simulink model "b_r309c_med"  (Simulink 6.2)
settings: Solver=ode45  StartTime=0.0  StopTime=1030.0  RelTol=1e-3
undefined symbols (not defined in the file): ant_bits, BEE2_usr, blockCountBits, blockRowBits, cmult_4bit_em
libraries: xbsIndex_r3 x2808, xps_library x97, casper_library x84
(part 3 of 20)

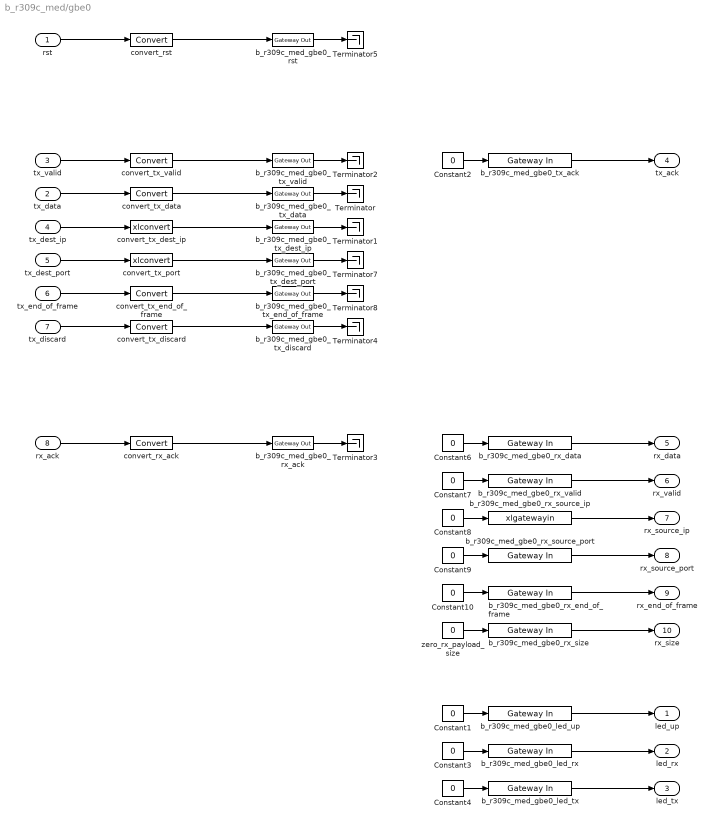
== system b_r309c_med/gbe0 ==
  rst : Inport  Port=1  LatchInput=off
  tx_data : Inport  Port=2  LatchInput=off
  tx_valid : Inport  Port=3  LatchInput=off
  tx_dest_ip : Inport  Port=4  LatchInput=off
  tx_dest_port : Inport  Port=5  LatchInput=off
  tx_end_of_frame : Inport  Port=6  LatchInput=off
  tx_discard : Inport  Port=7  LatchInput=off
  rx_ack : Inport  Port=8  LatchInput=off
  Constant{1..4,6..10} (9 alike) : Constant  Value=0
  Terminator{,1..5,7..8} (8 alike) : Terminator
  b_r309c_med_gbe0_led_rx : xbsIndex_r3/Gateway In  arith_type=Boolean  n_bits=1  bin_pt=0  quantization=Truncate  overflow=Wrap  period=1  timing_constraint=None  locs_specified=off  LOCs={}  needs_fixed_name=off  dbl_ovrd=off  show_param=off
      settings: xl_area=[0, 0, 0, 0, 0, 0, 0]
  b_r309c_med_gbe0_led_tx : xbsIndex_r3/Gateway In  arith_type=Boolean  n_bits=1  bin_pt=0  quantization=Truncate  overflow=Wrap  period=1  timing_constraint=None  locs_specified=off  LOCs={}  needs_fixed_name=off  dbl_ovrd=off  show_param=off
      settings: xl_area=[0, 0, 0, 0, 0, 0, 0]
  b_r309c_med_gbe0_led_up : xbsIndex_r3/Gateway In  arith_type=Boolean  n_bits=1  bin_pt=0  quantization=Truncate  overflow=Wrap  period=1  timing_constraint=None  locs_specified=off  LOCs={}  needs_fixed_name=off  dbl_ovrd=off  show_param=off
      settings: xl_area=[0, 0, 0, 0, 0, 0, 0]
  b_r309c_med_gbe0_rst : xbsIndex_r3/Gateway Out  output_type=Double  nbits=8  bin_pt=6  arith_type=Boolean  quantization=Truncate  overflow=Wrap  hdl_port=on  timing_constraint=None  locs_specified=off  LOCs={}  needs_fixed_name=off  show_param=off
      settings: xl_area=[0, 0, 0, 0, 0, 0, 0]
  b_r309c_med_gbe0_rx_ack : xbsIndex_r3/Gateway Out  output_type=Double  nbits=8  bin_pt=6  arith_type=Boolean  quantization=Truncate  overflow=Wrap  hdl_port=on  timing_constraint=None  locs_specified=off  LOCs={}  needs_fixed_name=off  show_param=off
      settings: xl_area=[0, 0, 0, 0, 0, 0, 0]
  b_r309c_med_gbe0_rx_data : xbsIndex_r3/Gateway In  arith_type=Unsigned  n_bits=64  bin_pt=0  quantization=Truncate  overflow=Wrap  period=1  timing_constraint=None  locs_specified=off  LOCs={}  needs_fixed_name=off  dbl_ovrd=off  show_param=off
      settings: xl_area=[0, 0, 0, 0, 0, 0, 0]
  b_r309c_med_gbe0_rx_end_of_frame : xbsIndex_r3/Gateway In  arith_type=Boolean  n_bits=1  bin_pt=0  quantization=Truncate  overflow=Wrap  period=1  timing_constraint=None  locs_specified=off  LOCs={}  needs_fixed_name=off  dbl_ovrd=off  show_param=off
      settings: xl_area=[0, 0, 0, 0, 0, 0, 0]
  b_r309c_med_gbe0_rx_size : xbsIndex_r3/Gateway In  arith_type=Unsigned  n_bits=16  bin_pt=0  quantization=Truncate  overflow=Wrap  period=1  timing_constraint=None  locs_specified=off  LOCs={}  needs_fixed_name=off  dbl_ovrd=off  show_param=off
      settings: xl_area=[0, 0, 0, 0, 0, 0, 0]
  b_r309c_med_gbe0_rx_source_ip : S-Function  AncestorBlock=xbsIndex_r3/Gateway In  FunctionName=xlgatewayin  Parameters="arith_type, n_bits, bin_pt, quantization, overflow,  gcb, period, dbl_ovrd, locs_specified, LOCs, timing_constraint, simulinkPeriod, designRoot, 0"  mask(Xilinx Gateway In){arith_type=Unsigned, n_bits=32, bin_pt=0, quantization=Truncate, overflow=Wrap, period=1, timing_constraint=None, locs_specified=off, LOCs={}, needs_fixed_name=off, dbl_ovrd=off, show_param=off, xl_area=[0, 0, 0, 0, 0, 0, 0], xl_use_area=off}
      mask prompts: arith_type "Output Data Type"; n_bits "Number of Bits"; bin_pt "Binary Point"; period "Sample Period"; timing_constraint "IOB Timing Constraint"; locs_specified "Specify IOB Location Constraints"; LOCs "IOB Pad Locations (specify as cell array {'MSB', ..., 'LSB'})"; needs_fixed_name "Do Not Prepend Hierarchy to Port Name"; dbl_ovrd "Override with Double"; show_param "---------------------- Show Implementation Parameters -----------------------------------------------------------------------------------"; xl_area "FPGA Area [Slices, FFs, BRAMs, LUTs, IOBs, Emb. Mults, TBUFs]"; xl_use_area "Use Area Above For Estimation"
      mask help:
      | Gateway in block.  Converts inputs of type Simulink integer, double and fixed point to  Xilinx fixed point type.
      |
      | Hardware notes:  In hardware these blocks become top level input ports.
      mask init:
      | [designRoot, family, part, speed, package, simulinkPeriod, sysclkPeriod, dbl_ovrd, trimVbit] = xlSysgenSettings(gcb,1,0);
      | trimVbit = 1;
      | [bg,fg] = xlcmap('IO',dbl_ovrd);
      | iPos = get_param(gcb,'Position');
      | iWidth=iPos(3)-iPos(1); iHeight=iPos(4)-iPos(2);
      | iCx=iWidth/2;
      | iCy=iHeight/2;
      | [logoX, logoY] = xlogo(iPos);
      mask Help: eval('xlWeb(xlhtmldoclink(''Gateway In''))');
      mask StyleString: popup(Boolean|Unsigned|Signed  (2's comp)),edit,edit,popup(Truncate|Round  (unbiased: +/- Inf)),popup(Wrap|Saturate|Flag as Error),edit,popup(None|Data Rate|Data Rate;  Set 'FAST' Attribute),checkbox,edit,checkbox,checkbox,checkbox,edit,checkbox
      mask CallbackString: xlgatewayinCallback|||||||xlgatewayinCallback||||xlShowIPCallback||
      mask Display:
      | patch([0 iWidth iWidth 0],[0 0 iHeight iHeight] , bg);
      | patch(logoX,logoY , fg);
      | port_label('input',1,'dbl');
      | port_label('output',1,'fpt');
      | 
      | ;plot([0 0 iWidth iWidth 0], [0 iHeight iHeight 0 0]);
  b_r309c_med_gbe0_rx_source_port : xbsIndex_r3/Gateway In  arith_type=Unsigned  n_bits=16  bin_pt=0  quantization=Truncate  overflow=Wrap  period=1  timing_constraint=None  locs_specified=off  LOCs={}  needs_fixed_name=off  dbl_ovrd=off  show_param=off
      settings: xl_area=[0, 0, 0, 0, 0, 0, 0]
  b_r309c_med_gbe0_rx_valid : xbsIndex_r3/Gateway In  arith_type=Boolean  n_bits=1  bin_pt=0  quantization=Truncate  overflow=Wrap  period=1  timing_constraint=None  locs_specified=off  LOCs={}  needs_fixed_name=off  dbl_ovrd=off  show_param=off
      settings: xl_area=[0, 0, 0, 0, 0, 0, 0]
  b_r309c_med_gbe0_tx_ack : xbsIndex_r3/Gateway In  arith_type=Boolean  n_bits=1  bin_pt=0  quantization=Truncate  overflow=Wrap  period=1  timing_constraint=None  locs_specified=off  LOCs={}  needs_fixed_name=off  dbl_ovrd=off  show_param=off
      settings: xl_area=[0, 0, 0, 0, 0, 0, 0]
  b_r309c_med_gbe0_tx_data : xbsIndex_r3/Gateway Out  output_type=Double  nbits=8  bin_pt=6  arith_type=Boolean  quantization=Truncate  overflow=Wrap  hdl_port=on  timing_constraint=None  locs_specified=off  LOCs={}  needs_fixed_name=off  show_param=off
      settings: xl_area=[0, 0, 0, 0, 0, 0, 0]
  b_r309c_med_gbe0_tx_dest_ip : xbsIndex_r3/Gateway Out  output_type=Double  nbits=8  bin_pt=6  arith_type=Boolean  quantization=Truncate  overflow=Wrap  hdl_port=on  timing_constraint=None  locs_specified=off  LOCs={}  needs_fixed_name=off  show_param=off
      settings: xl_area=[0, 0, 0, 0, 0, 0, 0]
  b_r309c_med_gbe0_tx_dest_port : xbsIndex_r3/Gateway Out  output_type=Double  nbits=8  bin_pt=6  arith_type=Boolean  quantization=Truncate  overflow=Wrap  hdl_port=on  timing_constraint=None  locs_specified=off  LOCs={}  needs_fixed_name=off  show_param=off
      settings: xl_area=[0, 0, 0, 0, 0, 0, 0]
  b_r309c_med_gbe0_tx_discard : xbsIndex_r3/Gateway Out  output_type=Double  nbits=8  bin_pt=6  arith_type=Boolean  quantization=Truncate  overflow=Wrap  hdl_port=on  timing_constraint=None  locs_specified=off  LOCs={}  needs_fixed_name=off  show_param=off
      settings: xl_area=[0, 0, 0, 0, 0, 0, 0]
  b_r309c_med_gbe0_tx_end_of_frame : xbsIndex_r3/Gateway Out  output_type=Double  nbits=8  bin_pt=6  arith_type=Boolean  quantization=Truncate  overflow=Wrap  hdl_port=on  timing_constraint=None  locs_specified=off  LOCs={}  needs_fixed_name=off  show_param=off
      settings: xl_area=[0, 0, 0, 0, 0, 0, 0]
  b_r309c_med_gbe0_tx_valid : xbsIndex_r3/Gateway Out  output_type=Double  nbits=8  bin_pt=6  arith_type=Boolean  quantization=Truncate  overflow=Wrap  hdl_port=on  timing_constraint=None  locs_specified=off  LOCs={}  needs_fixed_name=off  show_param=off
      settings: xl_area=[0, 0, 0, 0, 0, 0, 0]
  convert_rst : xbsIndex_r3/Convert  arith_type=Boolean  n_bits=64  bin_pt=0  quantization=Truncate  overflow=Wrap  latency=0  explicit_period=off  period=1  dbl_ovrd=off  show_param=off  inserted_by_tool=off  pipeline=off
      settings: xl_area=[0, 0, 0, 0, 0, 0, 0]
  convert_rx_ack : xbsIndex_r3/Convert  arith_type=Boolean  n_bits=64  bin_pt=0  quantization=Truncate  overflow=Wrap  latency=0  explicit_period=off  period=1  dbl_ovrd=off  show_param=off  inserted_by_tool=off  pipeline=off
      settings: xl_area=[0, 0, 0, 0, 0, 0, 0]
  convert_tx_data : xbsIndex_r3/Convert  arith_type=Unsigned  n_bits=64  bin_pt=0  quantization=Truncate  overflow=Wrap  latency=0  explicit_period=off  period=1  dbl_ovrd=off  show_param=off  inserted_by_tool=off  pipeline=off
      settings: xl_area=[0, 0, 0, 0, 0, 0, 0]
  convert_tx_dest_ip : S-Function  AncestorBlock=xbsIndex_r3/Convert  FunctionName=xlconvert  Parameters=sfcn_mwsv__  mask(Xilinx Converter Block){arith_type=Unsigned, n_bits=32, bin_pt=0, quantization=Truncate, overflow=Wrap, latency=0, explicit_period=off, period=1, dbl_ovrd=off, show_param=off, inserted_by_tool=off, pipeline=off, xl_area=[0, 0, 0, 0, 0, 0, 0], xl_use_area=off}
      mask prompts: arith_type "Output Type"; n_bits "Number of Bits"; bin_pt "Binary Point"; quantization "Quantization Behavior"; overflow "Overflow Behavior"; explicit_period "Use Explicit Sample Period"; period "Sample Period"; dbl_ovrd "Override with Doubles"; show_param "---------------------- Show Implementation Parameters -----------------------------------------------------------------------------------"; inserted_by_tool "Hidden Parameter:  inserted_by_tool"; pipeline "Pipeline to Greatest Extent Possible"; xl_area "FPGA Area [Slices, FFs, BRAMs, LUTs, IOBs, Emb. Mults, TBUFs]"; xl_use_area "Use Area Above For Estimation"
      mask help:
      | Type conversion block. The input is presented at the output after quantization and overflow effects.
      |
      | Hardware notes: Additional hardware is used when rounding or saturation is selected and output width is less than the input width.
      mask init:
      | [designRoot, family, part, speed, package, simulinkPeriod, sysclkPeriod, dbl_ovrd, trimVbit] = xlSysgenSettings(gcb,1,1);
      | if (arith_type==1)
      |   bool = 1;
      | else
      |   bool = 0;
      |   arith_type = arith_type-1;
      | end
      | zstr=''; zpstr='';
      | if latency > 0
      |   zstr = 'z';
      |   zpstr = sprintf('-%d', latency);
      | end
      | [bg,fg] = xlcmap('XBlock',dbl_ovrd);
      | if (inserted_by_tool)
      |   bg = [1.00 0.50 0.25];
      | end
      | iPos = get_param(gcb,'Position');
      | iWidth=iPos(3)-iPos(1); iHeight=iPos(4)-iPos(2);
      | iCx=iWidth/2;
      | iCy=iHeight/2;
      | [logoX, logoY] = xlogo(iPos);
      | zstrx = 0.45*iWidth-11; if (zstrx<3) zstrx=3; end
      | zstry = 0.36*iHeight-7; if (zstry<3) zstry=3; end
      | 
      | 
      | % one time added for param list
      | dblOvrd = dbl_ovrd;
      | precision0 = 2;
      | z0 = [n_bits bin_pt arith_type quantization overflow];
      | explicitClk = explicit_period;
      | 
      | 
      | % just pass everything to s-function
      | sfcn_mwsv__ = get_param(gcb, 'MaskWSVariables');
      mask Help: eval('xlWeb(xlhtmldoclink(''Convert''))');
      mask StyleString: popup(Boolean|Unsigned|Signed  (2's comp)),edit,edit,popup(Truncate|Round  (unbiased: +/- Inf)|Round  (unbiased: Even Values)),popup(Wrap|Saturate|Error),edit,checkbox,edit,checkbox,checkbox,checkbox,checkbox,edit,checkbox
      mask CallbackString: xlconvertCallback||||||xlMagicCallback|||xlShowIPCallback||||
      mask Display:
      | patch([0 iWidth iWidth 0],[0 0 iHeight iHeight] , bg);
      | patch(logoX,logoY , fg);
      | text(zstrx,zstry,zstr);
      | text(zstrx+5,zstry+5,zpstr);
      | port_label('output',1,'cast');
      | plot([0 0 iWidth iWidth 0], [0 iHeight iHeight 0 0]);
  convert_tx_discard : xbsIndex_r3/Convert  arith_type=Boolean  n_bits=1  bin_pt=0  quantization=Truncate  overflow=Wrap  latency=0  explicit_period=off  period=1  dbl_ovrd=off  show_param=off  inserted_by_tool=off  pipeline=off
      settings: xl_area=[0, 0, 0, 0, 0, 0, 0]
  convert_tx_end_of_frame : xbsIndex_r3/Convert  arith_type=Boolean  n_bits=1  bin_pt=0  quantization=Truncate  overflow=Wrap  latency=0  explicit_period=off  period=1  dbl_ovrd=off  show_param=off  inserted_by_tool=off  pipeline=off
      settings: xl_area=[0, 0, 0, 0, 0, 0, 0]
  convert_tx_port : S-Function  AncestorBlock=xbsIndex_r3/Convert  FunctionName=xlconvert  Parameters=sfcn_mwsv__  mask(Xilinx Converter Block){arith_type=Unsigned, n_bits=16, bin_pt=0, quantization=Truncate, overflow=Wrap, latency=0, explicit_period=off, period=1, dbl_ovrd=off, show_param=off, inserted_by_tool=off, pipeline=off, xl_area=[0, 0, 0, 0, 0, 0, 0], xl_use_area=off}
      mask prompts: arith_type "Output Type"; n_bits "Number of Bits"; bin_pt "Binary Point"; quantization "Quantization Behavior"; overflow "Overflow Behavior"; explicit_period "Use Explicit Sample Period"; period "Sample Period"; dbl_ovrd "Override with Doubles"; show_param "---------------------- Show Implementation Parameters -----------------------------------------------------------------------------------"; inserted_by_tool "Hidden Parameter:  inserted_by_tool"; pipeline "Pipeline to Greatest Extent Possible"; xl_area "FPGA Area [Slices, FFs, BRAMs, LUTs, IOBs, Emb. Mults, TBUFs]"; xl_use_area "Use Area Above For Estimation"
      mask help:
      | Type conversion block. The input is presented at the output after quantization and overflow effects.
      |
      | Hardware notes: Additional hardware is used when rounding or saturation is selected and output width is less than the input width.
      mask init: same as b_r309c_med/gbe0/convert_tx_dest_ip
      mask Help: eval('xlWeb(xlhtmldoclink(''Convert''))');
      mask StyleString: popup(Boolean|Unsigned|Signed  (2's comp)),edit,edit,popup(Truncate|Round  (unbiased: +/- Inf)|Round  (unbiased: Even Values)),popup(Wrap|Saturate|Error),edit,checkbox,edit,checkbox,checkbox,checkbox,checkbox,edit,checkbox
      mask CallbackString: xlconvertCallback||||||xlMagicCallback|||xlShowIPCallback||||
      mask Display:
      | patch([0 iWidth iWidth 0],[0 0 iHeight iHeight] , bg);
      | patch(logoX,logoY , fg);
      | text(zstrx,zstry,zstr);
      | text(zstrx+5,zstry+5,zpstr);
      | port_label('output',1,'cast');
      | plot([0 0 iWidth iWidth 0], [0 iHeight iHeight 0 0]);
  convert_tx_valid : xbsIndex_r3/Convert  arith_type=Boolean  n_bits=1  bin_pt=0  quantization=Truncate  overflow=Wrap  latency=0  explicit_period=off  period=1  dbl_ovrd=off  show_param=off  inserted_by_tool=off  pipeline=off
      settings: xl_area=[0, 0, 0, 0, 0, 0, 0]
  zero_rx_payload_size : Constant  Value=0
  led_up : Outport
  led_rx : Outport  Port=2
  led_tx : Outport  Port=3
  tx_ack : Outport  Port=4
  rx_data : Outport  Port=5
  rx_valid : Outport  Port=6
  rx_source_ip : Outport  Port=7
  rx_source_port : Outport  Port=8
  rx_end_of_frame : Outport  Port=9
  rx_size : Outport  Port=10
  wires:
  b_r309c_med_gbe0_tx_discard/1 -> Terminator4/1
  convert_tx_discard/1 -> b_r309c_med_gbe0_tx_discard/1
  tx_discard/1 -> convert_tx_discard/1
  b_r309c_med_gbe0_rx_size/1 -> rx_size/1
  zero_rx_payload_size/1 -> b_r309c_med_gbe0_rx_size/1
  b_r309c_med_gbe0_led_tx/1 -> led_tx/1
  Constant4/1 -> b_r309c_med_gbe0_led_tx/1
  b_r309c_med_gbe0_led_rx/1 -> led_rx/1
  Constant3/1 -> b_r309c_med_gbe0_led_rx/1
  b_r309c_med_gbe0_led_up/1 -> led_up/1
  Constant1/1 -> b_r309c_med_gbe0_led_up/1
  b_r309c_med_gbe0_rx_end_of_frame/1 -> rx_end_of_frame/1
  Constant10/1 -> b_r309c_med_gbe0_rx_end_of_frame/1
  b_r309c_med_gbe0_rx_source_port/1 -> rx_source_port/1
  Constant9/1 -> b_r309c_med_gbe0_rx_source_port/1
  Constant8/1 -> b_r309c_med_gbe0_rx_source_ip/1
  b_r309c_med_gbe0_rx_source_ip/1 -> rx_source_ip/1
  b_r309c_med_gbe0_tx_end_of_frame/1 -> Terminator8/1
  convert_tx_end_of_frame/1 -> b_r309c_med_gbe0_tx_end_of_frame/1
  tx_end_of_frame/1 -> convert_tx_end_of_frame/1
  b_r309c_med_gbe0_tx_dest_port/1 -> Terminator7/1
  convert_tx_port/1 -> b_r309c_med_gbe0_tx_dest_port/1
  tx_dest_port/1 -> convert_tx_port/1
  b_r309c_med_gbe0_rst/1 -> Terminator5/1
  convert_rst/1 -> b_r309c_med_gbe0_rst/1
  rst/1 -> convert_rst/1
  b_r309c_med_gbe0_rx_valid/1 -> rx_valid/1
  Constant7/1 -> b_r309c_med_gbe0_rx_valid/1
  b_r309c_med_gbe0_rx_ack/1 -> Terminator3/1
  Constant6/1 -> b_r309c_med_gbe0_rx_data/1
  Constant2/1 -> b_r309c_med_gbe0_tx_ack/1
  b_r309c_med_gbe0_tx_valid/1 -> Terminator2/1
  b_r309c_med_gbe0_tx_dest_ip/1 -> Terminator1/1
  b_r309c_med_gbe0_tx_data/1 -> Terminator/1
  b_r309c_med_gbe0_tx_ack/1 -> tx_ack/1
  convert_tx_valid/1 -> b_r309c_med_gbe0_tx_valid/1
  tx_valid/1 -> convert_tx_valid/1
  convert_tx_dest_ip/1 -> b_r309c_med_gbe0_tx_dest_ip/1
  tx_dest_ip/1 -> convert_tx_dest_ip/1
  convert_tx_data/1 -> b_r309c_med_gbe0_tx_data/1
  tx_data/1 -> convert_tx_data/1
  b_r309c_med_gbe0_rx_data/1 -> rx_data/1
  convert_rx_ack/1 -> b_r309c_med_gbe0_rx_ack/1
  rx_ack/1 -> convert_rx_ack/1

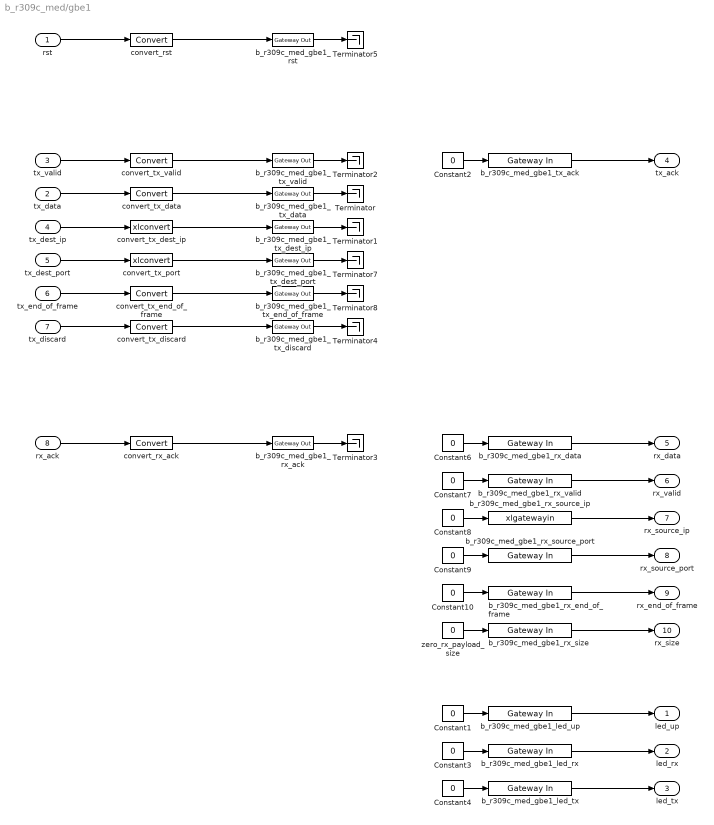
== system b_r309c_med/gbe1 ==
  rst : Inport  Port=1  LatchInput=off
  tx_data : Inport  Port=2  LatchInput=off
  tx_valid : Inport  Port=3  LatchInput=off
  tx_dest_ip : Inport  Port=4  LatchInput=off
  tx_dest_port : Inport  Port=5  LatchInput=off
  tx_end_of_frame : Inport  Port=6  LatchInput=off
  tx_discard : Inport  Port=7  LatchInput=off
  rx_ack : Inport  Port=8  LatchInput=off
  Constant{1..4,6..10} (9 alike) : Constant  Value=0
  Terminator{,1..5,7..8} (8 alike) : Terminator
  b_r309c_med_gbe1_led_rx : xbsIndex_r3/Gateway In  arith_type=Boolean  n_bits=1  bin_pt=0  quantization=Truncate  overflow=Wrap  period=1  timing_constraint=None  locs_specified=off  LOCs={}  needs_fixed_name=off  dbl_ovrd=off  show_param=off
      settings: xl_area=[0, 0, 0, 0, 0, 0, 0]
  b_r309c_med_gbe1_led_tx : xbsIndex_r3/Gateway In  arith_type=Boolean  n_bits=1  bin_pt=0  quantization=Truncate  overflow=Wrap  period=1  timing_constraint=None  locs_specified=off  LOCs={}  needs_fixed_name=off  dbl_ovrd=off  show_param=off
      settings: xl_area=[0, 0, 0, 0, 0, 0, 0]
  b_r309c_med_gbe1_led_up : xbsIndex_r3/Gateway In  arith_type=Boolean  n_bits=1  bin_pt=0  quantization=Truncate  overflow=Wrap  period=1  timing_constraint=None  locs_specified=off  LOCs={}  needs_fixed_name=off  dbl_ovrd=off  show_param=off
      settings: xl_area=[0, 0, 0, 0, 0, 0, 0]
  b_r309c_med_gbe1_rst : xbsIndex_r3/Gateway Out  output_type=Double  nbits=8  bin_pt=6  arith_type=Boolean  quantization=Truncate  overflow=Wrap  hdl_port=on  timing_constraint=None  locs_specified=off  LOCs={}  needs_fixed_name=off  show_param=off
      settings: xl_area=[0, 0, 0, 0, 0, 0, 0]
  b_r309c_med_gbe1_rx_ack : xbsIndex_r3/Gateway Out  output_type=Double  nbits=8  bin_pt=6  arith_type=Boolean  quantization=Truncate  overflow=Wrap  hdl_port=on  timing_constraint=None  locs_specified=off  LOCs={}  needs_fixed_name=off  show_param=off
      settings: xl_area=[0, 0, 0, 0, 0, 0, 0]
  b_r309c_med_gbe1_rx_data : xbsIndex_r3/Gateway In  arith_type=Unsigned  n_bits=64  bin_pt=0  quantization=Truncate  overflow=Wrap  period=1  timing_constraint=None  locs_specified=off  LOCs={}  needs_fixed_name=off  dbl_ovrd=off  show_param=off
      settings: xl_area=[0, 0, 0, 0, 0, 0, 0]
  b_r309c_med_gbe1_rx_end_of_frame : xbsIndex_r3/Gateway In  arith_type=Boolean  n_bits=1  bin_pt=0  quantization=Truncate  overflow=Wrap  period=1  timing_constraint=None  locs_specified=off  LOCs={}  needs_fixed_name=off  dbl_ovrd=off  show_param=off
      settings: xl_area=[0, 0, 0, 0, 0, 0, 0]
  b_r309c_med_gbe1_rx_size : xbsIndex_r3/Gateway In  arith_type=Unsigned  n_bits=16  bin_pt=0  quantization=Truncate  overflow=Wrap  period=1  timing_constraint=None  locs_specified=off  LOCs={}  needs_fixed_name=off  dbl_ovrd=off  show_param=off
      settings: xl_area=[0, 0, 0, 0, 0, 0, 0]
  b_r309c_med_gbe1_rx_source_ip : S-Function  AncestorBlock=xbsIndex_r3/Gateway In  FunctionName=xlgatewayin  Parameters="arith_type, n_bits, bin_pt, quantization, overflow,  gcb, period, dbl_ovrd, locs_specified, LOCs, timing_constraint, simulinkPeriod, designRoot, 0"  mask(Xilinx Gateway In){arith_type=Unsigned, n_bits=32, bin_pt=0, quantization=Truncate, overflow=Wrap, period=1, timing_constraint=None, locs_specified=off, LOCs={}, needs_fixed_name=off, dbl_ovrd=off, show_param=off, xl_area=[0, 0, 0, 0, 0, 0, 0], xl_use_area=off}
      mask prompts: arith_type "Output Data Type"; n_bits "Number of Bits"; bin_pt "Binary Point"; period "Sample Period"; timing_constraint "IOB Timing Constraint"; locs_specified "Specify IOB Location Constraints"; LOCs "IOB Pad Locations (specify as cell array {'MSB', ..., 'LSB'})"; needs_fixed_name "Do Not Prepend Hierarchy to Port Name"; dbl_ovrd "Override with Double"; show_param "---------------------- Show Implementation Parameters -----------------------------------------------------------------------------------"; xl_area "FPGA Area [Slices, FFs, BRAMs, LUTs, IOBs, Emb. Mults, TBUFs]"; xl_use_area "Use Area Above For Estimation"
      mask help:
      | Gateway in block.  Converts inputs of type Simulink integer, double and fixed point to  Xilinx fixed point type.
      |
      | Hardware notes:  In hardware these blocks become top level input ports.
      mask init: same as b_r309c_med/gbe0/b_r309c_med_gbe0_rx_source_ip
      mask Help: eval('xlWeb(xlhtmldoclink(''Gateway In''))');
      mask StyleString: popup(Boolean|Unsigned|Signed  (2's comp)),edit,edit,popup(Truncate|Round  (unbiased: +/- Inf)),popup(Wrap|Saturate|Flag as Error),edit,popup(None|Data Rate|Data Rate;  Set 'FAST' Attribute),checkbox,edit,checkbox,checkbox,checkbox,edit,checkbox
      mask CallbackString: xlgatewayinCallback|||||||xlgatewayinCallback||||xlShowIPCallback||
      mask Display:
      | patch([0 iWidth iWidth 0],[0 0 iHeight iHeight] , bg);
      | patch(logoX,logoY , fg);
      | port_label('input',1,'dbl');
      | port_label('output',1,'fpt');
      | 
      | ;plot([0 0 iWidth iWidth 0], [0 iHeight iHeight 0 0]);
  b_r309c_med_gbe1_rx_source_port : xbsIndex_r3/Gateway In  arith_type=Unsigned  n_bits=16  bin_pt=0  quantization=Truncate  overflow=Wrap  period=1  timing_constraint=None  locs_specified=off  LOCs={}  needs_fixed_name=off  dbl_ovrd=off  show_param=off
      settings: xl_area=[0, 0, 0, 0, 0, 0, 0]
  b_r309c_med_gbe1_rx_valid : xbsIndex_r3/Gateway In  arith_type=Boolean  n_bits=1  bin_pt=0  quantization=Truncate  overflow=Wrap  period=1  timing_constraint=None  locs_specified=off  LOCs={}  needs_fixed_name=off  dbl_ovrd=off  show_param=off
      settings: xl_area=[0, 0, 0, 0, 0, 0, 0]
  b_r309c_med_gbe1_tx_ack : xbsIndex_r3/Gateway In  arith_type=Boolean  n_bits=1  bin_pt=0  quantization=Truncate  overflow=Wrap  period=1  timing_constraint=None  locs_specified=off  LOCs={}  needs_fixed_name=off  dbl_ovrd=off  show_param=off
      settings: xl_area=[0, 0, 0, 0, 0, 0, 0]
  b_r309c_med_gbe1_tx_data : xbsIndex_r3/Gateway Out  output_type=Double  nbits=8  bin_pt=6  arith_type=Boolean  quantization=Truncate  overflow=Wrap  hdl_port=on  timing_constraint=None  locs_specified=off  LOCs={}  needs_fixed_name=off  show_param=off
      settings: xl_area=[0, 0, 0, 0, 0, 0, 0]
  b_r309c_med_gbe1_tx_dest_ip : xbsIndex_r3/Gateway Out  output_type=Double  nbits=8  bin_pt=6  arith_type=Boolean  quantization=Truncate  overflow=Wrap  hdl_port=on  timing_constraint=None  locs_specified=off  LOCs={}  needs_fixed_name=off  show_param=off
      settings: xl_area=[0, 0, 0, 0, 0, 0, 0]
  b_r309c_med_gbe1_tx_dest_port : xbsIndex_r3/Gateway Out  output_type=Double  nbits=8  bin_pt=6  arith_type=Boolean  quantization=Truncate  overflow=Wrap  hdl_port=on  timing_constraint=None  locs_specified=off  LOCs={}  needs_fixed_name=off  show_param=off
      settings: xl_area=[0, 0, 0, 0, 0, 0, 0]
  b_r309c_med_gbe1_tx_discard : xbsIndex_r3/Gateway Out  output_type=Double  nbits=8  bin_pt=6  arith_type=Boolean  quantization=Truncate  overflow=Wrap  hdl_port=on  timing_constraint=None  locs_specified=off  LOCs={}  needs_fixed_name=off  show_param=off
      settings: xl_area=[0, 0, 0, 0, 0, 0, 0]
  b_r309c_med_gbe1_tx_end_of_frame : xbsIndex_r3/Gateway Out  output_type=Double  nbits=8  bin_pt=6  arith_type=Boolean  quantization=Truncate  overflow=Wrap  hdl_port=on  timing_constraint=None  locs_specified=off  LOCs={}  needs_fixed_name=off  show_param=off
      settings: xl_area=[0, 0, 0, 0, 0, 0, 0]
  b_r309c_med_gbe1_tx_valid : xbsIndex_r3/Gateway Out  output_type=Double  nbits=8  bin_pt=6  arith_type=Boolean  quantization=Truncate  overflow=Wrap  hdl_port=on  timing_constraint=None  locs_specified=off  LOCs={}  needs_fixed_name=off  show_param=off
      settings: xl_area=[0, 0, 0, 0, 0, 0, 0]
  convert_rst : xbsIndex_r3/Convert  arith_type=Boolean  n_bits=64  bin_pt=0  quantization=Truncate  overflow=Wrap  latency=0  explicit_period=off  period=1  dbl_ovrd=off  show_param=off  inserted_by_tool=off  pipeline=off
      settings: xl_area=[0, 0, 0, 0, 0, 0, 0]
  convert_rx_ack : xbsIndex_r3/Convert  arith_type=Boolean  n_bits=64  bin_pt=0  quantization=Truncate  overflow=Wrap  latency=0  explicit_period=off  period=1  dbl_ovrd=off  show_param=off  inserted_by_tool=off  pipeline=off
      settings: xl_area=[0, 0, 0, 0, 0, 0, 0]
  convert_tx_data : xbsIndex_r3/Convert  arith_type=Unsigned  n_bits=64  bin_pt=0  quantization=Truncate  overflow=Wrap  latency=0  explicit_period=off  period=1  dbl_ovrd=off  show_param=off  inserted_by_tool=off  pipeline=off
      settings: xl_area=[0, 0, 0, 0, 0, 0, 0]
  convert_tx_dest_ip : S-Function  AncestorBlock=xbsIndex_r3/Convert  FunctionName=xlconvert  Parameters=sfcn_mwsv__  mask(Xilinx Converter Block){arith_type=Unsigned, n_bits=32, bin_pt=0, quantization=Truncate, overflow=Wrap, latency=0, explicit_period=off, period=1, dbl_ovrd=off, show_param=off, inserted_by_tool=off, pipeline=off, xl_area=[0, 0, 0, 0, 0, 0, 0], xl_use_area=off}
      mask prompts: arith_type "Output Type"; n_bits "Number of Bits"; bin_pt "Binary Point"; quantization "Quantization Behavior"; overflow "Overflow Behavior"; explicit_period "Use Explicit Sample Period"; period "Sample Period"; dbl_ovrd "Override with Doubles"; show_param "---------------------- Show Implementation Parameters -----------------------------------------------------------------------------------"; inserted_by_tool "Hidden Parameter:  inserted_by_tool"; pipeline "Pipeline to Greatest Extent Possible"; xl_area "FPGA Area [Slices, FFs, BRAMs, LUTs, IOBs, Emb. Mults, TBUFs]"; xl_use_area "Use Area Above For Estimation"
      mask help:
      | Type conversion block. The input is presented at the output after quantization and overflow effects.
      |
      | Hardware notes: Additional hardware is used when rounding or saturation is selected and output width is less than the input width.
      mask init: same as b_r309c_med/gbe0/convert_tx_dest_ip
      mask Help: eval('xlWeb(xlhtmldoclink(''Convert''))');
      mask StyleString: popup(Boolean|Unsigned|Signed  (2's comp)),edit,edit,popup(Truncate|Round  (unbiased: +/- Inf)|Round  (unbiased: Even Values)),popup(Wrap|Saturate|Error),edit,checkbox,edit,checkbox,checkbox,checkbox,checkbox,edit,checkbox
      mask CallbackString: xlconvertCallback||||||xlMagicCallback|||xlShowIPCallback||||
      mask Display:
      | patch([0 iWidth iWidth 0],[0 0 iHeight iHeight] , bg);
      | patch(logoX,logoY , fg);
      | text(zstrx,zstry,zstr);
      | text(zstrx+5,zstry+5,zpstr);
      | port_label('output',1,'cast');
      | plot([0 0 iWidth iWidth 0], [0 iHeight iHeight 0 0]);
  convert_tx_discard : xbsIndex_r3/Convert  arith_type=Boolean  n_bits=1  bin_pt=0  quantization=Truncate  overflow=Wrap  latency=0  explicit_period=off  period=1  dbl_ovrd=off  show_param=off  inserted_by_tool=off  pipeline=off
      settings: xl_area=[0, 0, 0, 0, 0, 0, 0]
  convert_tx_end_of_frame : xbsIndex_r3/Convert  arith_type=Boolean  n_bits=1  bin_pt=0  quantization=Truncate  overflow=Wrap  latency=0  explicit_period=off  period=1  dbl_ovrd=off  show_param=off  inserted_by_tool=off  pipeline=off
      settings: xl_area=[0, 0, 0, 0, 0, 0, 0]
  convert_tx_port : S-Function  AncestorBlock=xbsIndex_r3/Convert  FunctionName=xlconvert  Parameters=sfcn_mwsv__  mask(Xilinx Converter Block){arith_type=Unsigned, n_bits=16, bin_pt=0, quantization=Truncate, overflow=Wrap, latency=0, explicit_period=off, period=1, dbl_ovrd=off, show_param=off, inserted_by_tool=off, pipeline=off, xl_area=[0, 0, 0, 0, 0, 0, 0], xl_use_area=off}
      mask prompts: arith_type "Output Type"; n_bits "Number of Bits"; bin_pt "Binary Point"; quantization "Quantization Behavior"; overflow "Overflow Behavior"; explicit_period "Use Explicit Sample Period"; period "Sample Period"; dbl_ovrd "Override with Doubles"; show_param "---------------------- Show Implementation Parameters -----------------------------------------------------------------------------------"; inserted_by_tool "Hidden Parameter:  inserted_by_tool"; pipeline "Pipeline to Greatest Extent Possible"; xl_area "FPGA Area [Slices, FFs, BRAMs, LUTs, IOBs, Emb. Mults, TBUFs]"; xl_use_area "Use Area Above For Estimation"
      mask help:
      | Type conversion block. The input is presented at the output after quantization and overflow effects.
      |
      | Hardware notes: Additional hardware is used when rounding or saturation is selected and output width is less than the input width.
      mask init: same as b_r309c_med/gbe0/convert_tx_dest_ip
      mask Help: eval('xlWeb(xlhtmldoclink(''Convert''))');
      mask StyleString: popup(Boolean|Unsigned|Signed  (2's comp)),edit,edit,popup(Truncate|Round  (unbiased: +/- Inf)|Round  (unbiased: Even Values)),popup(Wrap|Saturate|Error),edit,checkbox,edit,checkbox,checkbox,checkbox,checkbox,edit,checkbox
      mask CallbackString: xlconvertCallback||||||xlMagicCallback|||xlShowIPCallback||||
      mask Display:
      | patch([0 iWidth iWidth 0],[0 0 iHeight iHeight] , bg);
      | patch(logoX,logoY , fg);
      | text(zstrx,zstry,zstr);
      | text(zstrx+5,zstry+5,zpstr);
      | port_label('output',1,'cast');
      | plot([0 0 iWidth iWidth 0], [0 iHeight iHeight 0 0]);
  convert_tx_valid : xbsIndex_r3/Convert  arith_type=Boolean  n_bits=1  bin_pt=0  quantization=Truncate  overflow=Wrap  latency=0  explicit_period=off  period=1  dbl_ovrd=off  show_param=off  inserted_by_tool=off  pipeline=off
      settings: xl_area=[0, 0, 0, 0, 0, 0, 0]
  zero_rx_payload_size : Constant  Value=0
  led_up : Outport
  led_rx : Outport  Port=2
  led_tx : Outport  Port=3
  tx_ack : Outport  Port=4
  rx_data : Outport  Port=5
  rx_valid : Outport  Port=6
  rx_source_ip : Outport  Port=7
  rx_source_port : Outport  Port=8
  rx_end_of_frame : Outport  Port=9
  rx_size : Outport  Port=10
  wires:
  b_r309c_med_gbe1_tx_discard/1 -> Terminator4/1
  convert_tx_discard/1 -> b_r309c_med_gbe1_tx_discard/1
  tx_discard/1 -> convert_tx_discard/1
  b_r309c_med_gbe1_rx_size/1 -> rx_size/1
  zero_rx_payload_size/1 -> b_r309c_med_gbe1_rx_size/1
  b_r309c_med_gbe1_led_tx/1 -> led_tx/1
  Constant4/1 -> b_r309c_med_gbe1_led_tx/1
  b_r309c_med_gbe1_led_rx/1 -> led_rx/1
  Constant3/1 -> b_r309c_med_gbe1_led_rx/1
  b_r309c_med_gbe1_led_up/1 -> led_up/1
  Constant1/1 -> b_r309c_med_gbe1_led_up/1
  b_r309c_med_gbe1_rx_end_of_frame/1 -> rx_end_of_frame/1
  Constant10/1 -> b_r309c_med_gbe1_rx_end_of_frame/1
  b_r309c_med_gbe1_rx_source_port/1 -> rx_source_port/1
  Constant9/1 -> b_r309c_med_gbe1_rx_source_port/1
  Constant8/1 -> b_r309c_med_gbe1_rx_source_ip/1
  b_r309c_med_gbe1_rx_source_ip/1 -> rx_source_ip/1
  b_r309c_med_gbe1_tx_end_of_frame/1 -> Terminator8/1
  convert_tx_end_of_frame/1 -> b_r309c_med_gbe1_tx_end_of_frame/1
  tx_end_of_frame/1 -> convert_tx_end_of_frame/1
  b_r309c_med_gbe1_tx_dest_port/1 -> Terminator7/1
  convert_tx_port/1 -> b_r309c_med_gbe1_tx_dest_port/1
  tx_dest_port/1 -> convert_tx_port/1
  b_r309c_med_gbe1_rst/1 -> Terminator5/1
  convert_rst/1 -> b_r309c_med_gbe1_rst/1
  rst/1 -> convert_rst/1
  b_r309c_med_gbe1_rx_valid/1 -> rx_valid/1
  Constant7/1 -> b_r309c_med_gbe1_rx_valid/1
  b_r309c_med_gbe1_rx_ack/1 -> Terminator3/1
  Constant6/1 -> b_r309c_med_gbe1_rx_data/1
  Constant2/1 -> b_r309c_med_gbe1_tx_ack/1
  b_r309c_med_gbe1_tx_valid/1 -> Terminator2/1
  b_r309c_med_gbe1_tx_dest_ip/1 -> Terminator1/1
  b_r309c_med_gbe1_tx_data/1 -> Terminator/1
  b_r309c_med_gbe1_tx_ack/1 -> tx_ack/1
  convert_tx_valid/1 -> b_r309c_med_gbe1_tx_valid/1
  tx_valid/1 -> convert_tx_valid/1
  convert_tx_dest_ip/1 -> b_r309c_med_gbe1_tx_dest_ip/1
  tx_dest_ip/1 -> convert_tx_dest_ip/1
  convert_tx_data/1 -> b_r309c_med_gbe1_tx_data/1
  tx_data/1 -> convert_tx_data/1
  b_r309c_med_gbe1_rx_data/1 -> rx_data/1
  convert_rx_ack/1 -> b_r309c_med_gbe1_rx_ack/1
  rx_ack/1 -> convert_rx_ack/1

== system b_r309c_med/loopback0 ==
  note: Only take packets transmitted
      | to my own IP address
  din : Inport  Port=1  LatchInput=off
  we : Inport  Port=2  LatchInput=off
  dest_ip : Inport  Port=3  LatchInput=off
  eof : Inport  Port=4  LatchInput=off
  discard : Inport  Port=5  LatchInput=off
  my_ip : Inport  Port=6  LatchInput=off
  ack : Inport  Port=7  LatchInput=off
  Concat : xbsIndex_r3/Concat  num_inputs=2  explicit_period=off  period=1  dbl_ovrd=off
  Constant1 : xbsIndex_r3/Constant  const=1  equ=P=C  arith_type=Boolean  n_bits=2  bin_pt=0  opselect=C  inp2=PCIN>>17  opr=+  inp1=P  carry=CIN  iostate=0  explicit_period=on  period=1  dbl_ovrd=off
  Convert : xbsIndex_r3/Convert  arith_type=Unsigned  n_bits=1  bin_pt=0  quantization=Truncate  overflow=Wrap  latency=0  explicit_period=off  period=1  dbl_ovrd=off  show_param=off  inserted_by_tool=off  pipeline=off
      settings: xl_area=[0, 0, 0, 0, 0, 0, 0]
  Inverter1 : xbsIndex_r3/Inverter  latency=0  explicit_period=off  period=1  en=off  dbl_ovrd=off  show_param=off
      settings: xl_area=[0, 0, 0, 0, 0, 0, 0]
  Logical1 : xbsIndex_r3/Logical  logical_function=OR  inputs=2  precision=Full  arith_type=Unsigned  n_bits=8  bin_pt=2  align_bp=on  latency=0  explicit_period=off  period=1  en=off  dbl_ovrd=off  show_param=off
      settings: xl_area=[0, 0, 0, 0, 0, 0, 0]
  Logical2 : xbsIndex_r3/Logical  logical_function=AND  inputs=2  precision=Full  arith_type=Unsigned  n_bits=8  bin_pt=2  align_bp=on  latency=0  explicit_period=off  period=1  en=off  dbl_ovrd=off  show_param=off
      settings: xl_area=[0, 0, 0, 0, 0, 0, 0]
  Logical4 : xbsIndex_r3/Logical  logical_function=AND  inputs=2  precision=Full  arith_type=Unsigned  n_bits=8  bin_pt=2  align_bp=on  latency=0  explicit_period=off  period=1  en=off  dbl_ovrd=off  show_param=off
      settings: xl_area=[0, 0, 0, 0, 0, 0, 0]
  Relational1 : xbsIndex_r3/Relational  mode=a=b  latency=1  explicit_period=off  period=1  en=off  dbl_ovrd=off  show_param=off
      settings: xl_area=[0, 0, 0, 0, 0, 0, 0]
  Slice : xbsIndex_r3/Slice  mode=Upper Bit Location + Width  nbits=1  bit1=0  base1=MSB of Input  bit0=0  base0=LSB of Input  boolean_output=on  explicit_period=off  period=1  dbl_ovrd=off
  Slice1 : xbsIndex_r3/Slice  mode=Lower Bit Location + Width  nbits=64  bit1=-1  base1=MSB of Input  bit0=0  base0=LSB of Input  boolean_output=off  explicit_period=off  period=1  dbl_ovrd=off
  fwft_fifo : Subsystem
  rollback_fifo : Subsystem  mask{depth_bits=depth_bits}
      mask prompts: depth_bits "Fifo Depth (2^?):"
      mask help: A rollback fifo behaves as a normal fifo, except that data which are written in have to be "committed" before they become available for readout. Moreover, any data which are written in and have not been committed can be "discarded", and will never be made available for readout.
  dout : Outport
  valid : Outport  Port=2
  eof_out : Outport  Port=3
  wires:
  Logical2/1 -> Logical1/1
  Inverter1/1 -> Logical2/2
  discard/1 -> Logical1/2
  Logical1/1 -> rollback_fifo/4(discard)
  Convert/1 -> Concat/1
  Slice/1 -> eof_out/1
  Slice1/1 -> dout/1
  din/1 -> Concat/2
  Concat/1 -> rollback_fifo/1(din)
  Logical4/1 -> rollback_fifo/3(commit)
  we/1 -> rollback_fifo/2(we)
  eof/1 -> Logical2/1, Logical4/1, Convert/1
  Relational1/1 -> Inverter1/1, Logical4/2
  my_ip/1 -> Relational1/2
  dest_ip/1 -> Relational1/1
  rollback_fifo/1(dout) -> fwft_fifo/1(din)
  rollback_fifo/2(valid) -> fwft_fifo/2(we)
  Constant1/1 -> rollback_fifo/5(re)
  ack/1 -> fwft_fifo/3(ack)
  fwft_fifo/1(dout) -> Slice1/1, Slice/1
  fwft_fifo/2(valid) -> valid/1

== system b_r309c_med/miss_cnt0 ==
  rst : Inport  Port=1  LatchInput=off
  valid : Inport  Port=2  LatchInput=off
  rcvd : Inport  Port=3  LatchInput=off
  Counter3 : xbsIndex_r3/Counter  cnt_type=Free Running  n_bits=32  bin_pt=0  arith_type=Unsigned  start_count=0  cnt_to=1023  cnt_by_val=1  operation=Up  explicit_period=on  period=1  load_pin=off  rst=on  en=on  dbl_ovrd=off  show_param=off  use_rpm=on  gen_core=off
      settings: xl_area=[0, 0, 0, 0, 0, 0, 0]
  Inverter : xbsIndex_r3/Inverter  latency=0  explicit_period=off  period=1  en=off  dbl_ovrd=off  show_param=off
      settings: xl_area=[0, 0, 0, 0, 0, 0, 0]
  Logical2 : xbsIndex_r3/Logical  logical_function=AND  inputs=2  precision=Full  arith_type=Unsigned  n_bits=8  bin_pt=2  align_bp=on  latency=0  explicit_period=on  period=1  en=off  dbl_ovrd=off  show_param=off
      settings: xl_area=[0, 0, 0, 0, 0, 0, 0]
  cnt : Outport
  wires:
  Logical2/1 -> Counter3/2
  rst/1 -> Counter3/1
  valid/1 -> Logical2/1
  Counter3/1 -> cnt/1
  rcvd/1 -> Inverter/1
  Inverter/1 -> Logical2/2

== system b_r309c_med/mux_pkts0 ==
  note: Read from loopback if a gbe packet
      | has been received with a higher mcnt.
      | Otherwise, wait until gbe has one ready.
      | Once packet readout begins, wait for eof
      | before choosing between gbe & loopback again.
  note: Register the first valid
      | data of a packet (mcnt)
      | from the gbe.
  note: Only take data from loopback
      | if a higher mcnt has been
      | received from gbe.
  gbe_din : Inport  Port=1  LatchInput=off
  gbe_valid : Inport  Port=2  LatchInput=off
  gbe_eof : Inport  Port=3  LatchInput=off
  loop_din : Inport  Port=4  LatchInput=off
  loop_valid : Inport  Port=5  LatchInput=off
  loop_eof : Inport  Port=6  LatchInput=off
  Concat2 : xbsIndex_r3/Concat  num_inputs=2  explicit_period=off  period=1  dbl_ovrd=off
  Constant1 : Constant  Value=0
  Convert : xbsIndex_r3/Convert  arith_type=Boolean  n_bits=8  bin_pt=6  quantization=Truncate  overflow=Wrap  latency=0  explicit_period=off  period=1  dbl_ovrd=off  show_param=off  inserted_by_tool=off  pipeline=off
      settings: xl_area=[0, 0, 0, 0, 0, 0, 0]
  Convert1 : xbsIndex_r3/Convert  arith_type=Boolean  n_bits=8  bin_pt=6  quantization=Truncate  overflow=Wrap  latency=0  explicit_period=off  period=1  dbl_ovrd=off  show_param=off  inserted_by_tool=off  pipeline=off
      settings: xl_area=[0, 0, 0, 0, 0, 0, 0]
  Convert2 : xbsIndex_r3/Convert  arith_type=Boolean  n_bits=8  bin_pt=6  quantization=Truncate  overflow=Wrap  latency=0  explicit_period=off  period=1  dbl_ovrd=off  show_param=off  inserted_by_tool=off  pipeline=off
      settings: xl_area=[0, 0, 0, 0, 0, 0, 0]
  Convert{4..5,7..8} (4 alike) : xbsIndex_r3/Convert  arith_type=Boolean  n_bits=1  bin_pt=0  quantization=Truncate  overflow=Wrap  latency=0  explicit_period=on  period=1  dbl_ovrd=off  show_param=off  inserted_by_tool=off  pipeline=off
      settings: xl_area=[0, 0, 0, 0, 0, 0, 0]
  Convert6 : xbsIndex_r3/Convert  arith_type=Unsigned  n_bits=1  bin_pt=0  quantization=Truncate  overflow=Wrap  latency=0  explicit_period=off  period=1  dbl_ovrd=off  show_param=off  inserted_by_tool=off  pipeline=off
      settings: xl_area=[0, 0, 0, 0, 0, 0, 0]
  Delay1 : xbsIndex_r3/Delay  latency=1  reg_retiming=off  explicit_period=off  period=1  en=off  accept_only_valid=off  init_zero=on  dbl_ovrd=off  show_param=off
      settings: xl_area=[0, 0, 0, 0, 0, 0, 0]
  Inverter2 : xbsIndex_r3/Inverter  Orientation=left  latency=0  explicit_period=off  period=1  en=off  dbl_ovrd=off  show_param=off
      settings: xl_area=[0, 0, 0, 0, 0, 0, 0]
  Logical : xbsIndex_r3/Logical  logical_function=OR  inputs=2  precision=Full  arith_type=Unsigned  n_bits=8  bin_pt=2  align_bp=on  latency=0  explicit_period=off  period=1  en=off  dbl_ovrd=off  show_param=off
      settings: xl_area=[0, 0, 0, 0, 0, 0, 0]
  Logical{1..5,7..8} (7 alike) : xbsIndex_r3/Logical  logical_function=AND  inputs=2  precision=Full  arith_type=Unsigned  n_bits=8  bin_pt=2  align_bp=on  latency=0  explicit_period=off  period=1  en=off  dbl_ovrd=off  show_param=off
      settings: xl_area=[0, 0, 0, 0, 0, 0, 0]
  Logical9 : xbsIndex_r3/Logical  logical_function=OR  inputs=2  precision=Full  arith_type=Unsigned  n_bits=8  bin_pt=2  align_bp=on  latency=1  explicit_period=off  period=1  en=off  dbl_ovrd=off  show_param=off
      settings: xl_area=[0, 0, 0, 0, 0, 0, 0]
  Mux : xbsIndex_r3/Mux  inputs=2  precision=Full  arith_type="Signed  (2's comp)"  n_bits=8  bin_pt=2  quantization=Truncate  overflow=Wrap  latency=1  explicit_period=off  period=1  en=off  dbl_ovrd=off  show_param=off  mux_type=off  use_rpm=off  gen_core=off
      settings: xl_area=[0, 0, 0, 0, 0, 0, 0]
  Mux2 : xbsIndex_r3/Mux  inputs=2  precision=Full  arith_type="Signed  (2's comp)"  n_bits=8  bin_pt=2  quantization=Truncate  overflow=Wrap  latency=0  explicit_period=off  period=1  en=off  dbl_ovrd=off  show_param=off  mux_type=off  use_rpm=off  gen_core=off
      settings: xl_area=[0, 0, 0, 0, 0, 0, 0]
  Relational1 : xbsIndex_r3/Relational  mode=a<=b  latency=1  explicit_period=off  period=1  en=off  dbl_ovrd=off  show_param=off
      settings: xl_area=[0, 0, 0, 0, 0, 0, 0]
  Slice : xbsIndex_r3/Slice  mode=Lower Bit Location + Width  nbits=1  bit1=0  base1=MSB of Input  bit0=1  base0=LSB of Input  boolean_output=off  explicit_period=off  period=1  dbl_ovrd=off
  Slice1 : xbsIndex_r3/Slice  mode=Upper Bit Location + Width  nbits=48  bit1=0  base1=MSB of Input  bit0=0  base0=LSB of Input  boolean_output=off  explicit_period=off  period=1  dbl_ovrd=off
  Slice2 : xbsIndex_r3/Slice  mode=Lower Bit Location + Width  nbits=16  bit1=0  base1=MSB of Input  bit0=0  base0=LSB of Input  boolean_output=off  explicit_period=off  period=1  dbl_ovrd=off
  Slice3 : xbsIndex_r3/Slice  mode=Upper Bit Location + Width  nbits=48  bit1=0  base1=MSB of Input  bit0=0  base0=LSB of Input  boolean_output=off  explicit_period=off  period=1  dbl_ovrd=off
  Slice4 : xbsIndex_r3/Slice  mode=Lower Bit Location + Width  nbits=16  bit1=0  base1=MSB of Input  bit0=0  base0=LSB of Input  boolean_output=off  explicit_period=off  period=1  dbl_ovrd=off
  Slice5 : xbsIndex_r3/Slice  mode=Lower Bit Location + Width  nbits=1  bit1=0  base1=MSB of Input  bit0=0  base0=LSB of Input  boolean_output=off  explicit_period=off  period=1  dbl_ovrd=off
  gbe_mcnt : xbsIndex_r3/Register  init=0  reg_only_valid=off  explicit_period=on  period=1  rst=on  en=on  out_en=off  dbl_ovrd=off  show_param=off
      settings: xl_area=[0, 0, 0, 0, 0, 0, 0]
  loop_mcnt : xbsIndex_r3/Register  init=0  reg_only_valid=off  explicit_period=on  period=1  rst=on  en=on  out_en=off  dbl_ovrd=off  show_param=off
      settings: xl_area=[0, 0, 0, 0, 0, 0, 0]
  mcnt : xps_library/software register  Tag=xps:sw_reg  io_dir=To Processor  arith_type=Unsigned  bitwidth=32  bin_pt=0  sample_period=1  gw_name=b_r309c_med_mux_pkts0_mcnt_user_data_in
  posedge : casper_library/Misc/posedge  Tag=Rising Edge Detector
  rst_mcnt_regs : xps_library/software register  Tag=xps:sw_reg  io_dir=From Processor  arith_type=Unsigned  bitwidth=32  bin_pt=0  sample_period=1  gw_name=b_r309c_med_mux_pkts0_rst_mcnt_regs_user_data_out
  state_mach : Subsystem
  dout : Outport
  valid : Outport  Port=2
  eof : Outport  Port=3
  loop_ack : Outport  Port=4
  gbe_ack : Outport  Port=5
  wires:
  Mux/1 -> dout/1
  Logical9/1 -> Convert/1
  Mux2/1 -> Delay1/1, state_mach/3(eof)
  Delay1/1 -> eof/1
  gbe_din/1 -> Mux/3, Slice1/1
  loop_din/1 -> Mux/2, Slice3/1
  gbe_valid/1 -> Convert8/1
  loop_valid/1 -> Convert4/1
  state_mach/1(gbe_ack) -> Mux2/1, Convert6/1, Logical8/1, Convert5/1
  gbe_eof/1 -> Logical1/2
  loop_eof/1 -> Logical4/2
  Logical4/1 -> Mux2/2
  Logical1/1 -> Mux2/3
  state_mach/2(loop_ack) -> Logical7/1, Convert7/1
  Convert/1 -> valid/1
  Slice1/1 -> gbe_mcnt/1
  state_mach/3(state) -> Inverter2/1
  Inverter2/1 -> Logical2/1, Logical5/1
  gbe_mcnt/1 -> Relational1/2, Slice4/1
  Relational1/1 -> Logical3/1
  loop_mcnt/1 -> Relational1/1, Slice2/1
  Slice3/1 -> loop_mcnt/1
  Slice2/1 -> Concat2/1
  Slice4/1 -> Concat2/2
  Concat2/1 -> mcnt/1
  Convert6/1 -> Mux/1
  Convert5/1 -> gbe_ack/1
  Convert7/1 -> loop_ack/1
  Convert4/1 -> Logical4/1, Logical3/2, Logical7/2, Logical5/2
  Convert8/1 -> Logical2/2, Logical1/1, state_mach/1(gbe_valid), Logical8/2
  Logical7/1 -> Logical9/1
  Logical8/1 -> Logical9/2
  Logical/1 -> state_mach/2(pkt_rdy)
  Logical3/1 -> Logical/1
  Logical2/1 -> gbe_mcnt/3
  Logical5/1 -> loop_mcnt/3
  Slice/1 -> Convert1/1
  Constant1/1 -> rst_mcnt_regs/1
  rst_mcnt_regs/1 -> Slice5/1, Slice/1
  Slice5/1 -> posedge/1
  posedge/1 -> Convert2/1
  Convert1/1 -> Logical/2
  Convert2/1 -> loop_mcnt/2, gbe_mcnt/2
